simulink model "Three_Phase_Diode_Rectifier"  (R2021b)
settings: Solver=VariableStepAuto  StartTime=0.0  StopTime=0.05  MaxStep=1e-5  RelTol=1e-3
libraries: spsDiodeLib x6, spsACVoltageSourceLib x3, spsCurrentMeasurementLib x2, spsVoltageMeasurementLib x2, spsMeanLib x1, spsSeriesRLCBranchLib x1, spsTHDLib x1, spspowerguiLib x1
settings Model: Creator=pc  LastModifiedBy=pc

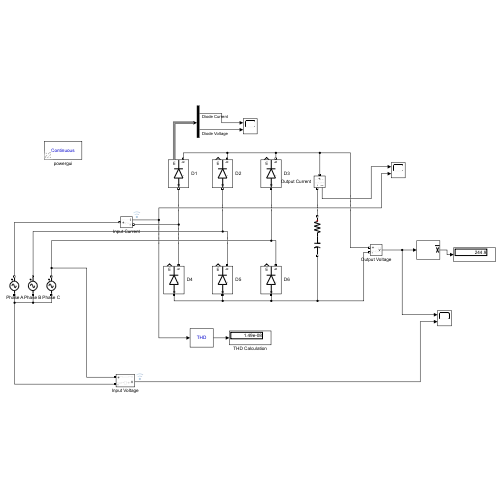
[thumbnail: Simulink's stored preview of the top-level diagram]
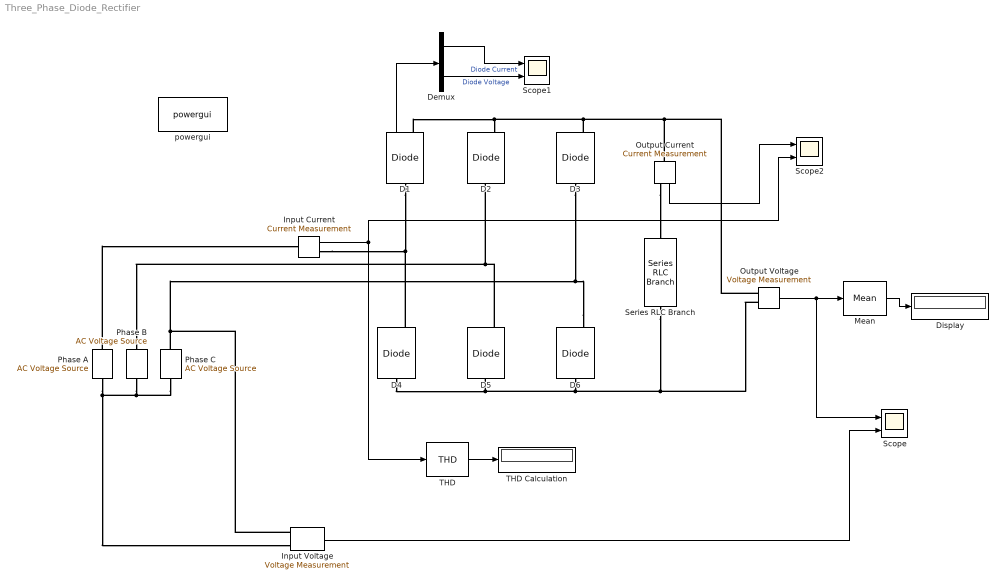
== system Three_Phase_Diode_Rectifier ==
  " Phase A" : spsACVoltageSourceLib/AC Voltage Source  Amplitude=100*sqrt(2)  Phase=0  Frequency=50  SampleTime=0  Measurements=None  BusType=swing  Pref=10e3  Qref=0  Qmin=-inf  Qmax=+inf
  D{1..6} (6 alike) : spsDiodeLib/Diode  Ron=0  Lon=0  Vf=0  IC=0  UseSnubber=0  Rs=inf  Cs=0  Measurements=on
  Demux : Demux  Outputs=2
  Display : Display
  Input Current : spsCurrentMeasurementLib/Current Measurement  PhasorSimulation=off  OutputType=Complex  PSBequivalent=0
  Input Voltage : spsVoltageMeasurementLib/Voltage Measurement  PhasorSimulation=off  OutputType=Complex  PSBequivalent=0
  Mean : spsMeanLib/Mean  Freq=50  Vinit=0  Ts=0
  Output Current : spsCurrentMeasurementLib/Current Measurement  PhasorSimulation=off  OutputType=Complex  PSBequivalent=0
  Output Voltage : spsVoltageMeasurementLib/Voltage Measurement  PhasorSimulation=off  OutputType=Complex  PSBequivalent=0
  Phase B : spsACVoltageSourceLib/AC Voltage Source  Amplitude=100*sqrt(2)  Phase=-120  Frequency=50  SampleTime=0  Measurements=None  BusType=swing  Pref=10e3  Qref=0  Qmin=-inf  Qmax=+inf
  Phase C : spsACVoltageSourceLib/AC Voltage Source  Amplitude=100*sqrt(2)  Phase=120  Frequency=50  SampleTime=0  Measurements=None  BusType=swing  Pref=10e3  Qref=0  Qmin=-inf  Qmax=+inf
  Scope : Scope  NumInputPorts=2
  Scope1 : Scope  NumInputPorts=2
  Scope2 : Scope  NumInputPorts=2
  Series RLC Branch : spsSeriesRLCBranchLib/Series RLC Branch  LConnTagsString=__new0  RConnTagsString=__new0  BranchType=RC  Resistance=1  Inductance=1e-3  SetiL0=off  InitialCurrent=0  Capacitance=1e-6  Setx0=off  InitialVoltage=0  Measurements=None
  THD : spsTHDLib/THD  Freq=60  Ts=0
      settings: SourceProductBaseCode=PS
  THD Calculation : Display
  powergui : spspowerguiLib/powergui  Priority=1  SimulationMode=Continuous  SampleTime=50e-6  frequency=60  Iterations=50  frequencyindice=50  Pbase=100e6  ErrMax=1e-4  UnitsV=kV  UnitsW=MW  buscounter=0  FunctionMessages=off  echomessages=off  EnableUseOfTLC=off  CurrentSourceSwitches=off  DisableSnubberDevices=off  DisableRonSwitches=off  DisableVfSwitches=off  DisplayEquations=off  AutomaticDiscreteSolvers=off  SolverType=Tustin/Backward Euler (TBE)  Interpol=off  ExternalGateDelay=off  methode=off  Ts=100  x0status=blocks  SPID=on  SwTol=0  HookPort=off  NonlinearTolerance=1e-4  nMaxIteration=100  ContinueOnMaxIteration=off  RestoreLinks=warning  ResistiveCurrentMeasurement=off  Frange=[0:2:500]  Ylog=off  Xlog=on  ShowGrid=off  save=off  variable=ZData  structure=0  ZoomFFT=off  StartTime=0.0  cycles=1  DisplayStyle=1  fundamental=60  FreqAxis=off  MaxFrequency=1000  frequencyindicesteady=1  RmsSteady=1  display=off
  wires:
  THD/1 -> THD Calculation/1
  Mean/1 -> Display/1
  Output Voltage/1 -> Scope/1, Mean/1
  Input Voltage/1 -> Scope/2
  D1/1 -> Demux/1
  Demux/1 -> Scope1/1  "Diode Current"
  Demux/2 -> Scope1/2  "Diode Voltage"
  Output Current/1 -> Scope2/1
  Input Current/1 -> THD/1, Scope2/2
  connections:
  D2/RConn1 -- Output Current/LConn1 -- Output Voltage/LConn1 -- D3/RConn1 -- D1/RConn1
  D6/RConn1 -- Input Voltage/LConn1 -- Phase C/RConn1 -- D3/LConn1
  D6/LConn1 -- Series RLC Branch/RConn1 -- Output Voltage/LConn2 -- D4/LConn1 -- D5/LConn1
  Input Current/RConn1 -- D1/LConn1 -- D4/RConn1
  D2/LConn1 -- Phase B/RConn1 -- D5/RConn1
  " Phase A"/RConn1 -- Input Current/LConn1
  " Phase A"/LConn1 -- Phase C/LConn1 -- Phase B/LConn1 -- Input Voltage/LConn2
  Output Current/RConn1 -- Series RLC Branch/LConn1
